simulink model "CtrPlatform"  (Simulink 7.9)
settings: Solver=ode3  StartTime=0.0  StopTime=8  FixedStep=Ts  RelTol=1e-3
InitFcn:
  | eval('CtrPlatformCfg')
StopFcn:
  | eval('CtrPlotTrj')
values from neighbouring files (symbols this model uses):
  A = [a1 a2 a3 a4 a5 a6]/180*pi    [Config.m]    (also in CtrPlatformCfg.m)
  a2 = 0    [Config.m]    (also in CtrPlatformCfg.m)
  a3 = 0    [Config.m]    (also in CtrPlatformCfg.m)
  a4 = 0    [Config.m]    (also in CtrPlatformCfg.m)
  a5 = 90    [Config.m]    (also in CtrPlatformCfg.m)
  a6 = 0    [Config.m]    (also in CtrPlatformCfg.m)
  Cen = Cen(:)'    [Config.m]    (also in CtrPlatformCfg.m; DynEulerTest.m = Cen'; EfDynCAD.m = [cen1,cen2,cen3,cen4,cen5,cen6]')
  CurPulseFreq = 0.25*2*pi    (= 1.57079632679)    [Config.m]    (also in CtrPlatformCfg.m)
  Deg2Rad = pi/180    (= 0.0174532925199)    [Config.m]    (also in CtrPlatformCfg.m)
  DisturbSelect = 2    [Config.m]    (also in CtrPlatformCfg.m)
  DynTrjMode = 3    [Config.m]    (also in CtrPlatformCfg.m = 1)
  FbDisturbSelect = 2    [Config.m]    (also in CtrPlatformCfg.m)
  freq = tvel/radius    (= 1)    [Config.m]    (also in CtrPlatformCfg.m)
  FrictionSelect = 2    [CtrPlatformCfg.m]
  Gravity = 9.8    [Config.m]    (also in CtrPlatformCfg.m)
  Ie1 = in1(:)'    [Config.m]    (also in CtrPlatformCfg.m; DynEulerTest.m = in1(:); EfDynCAD.m = in1(:))
  Ie2 = in2(:)'    [Config.m]    (also in CtrPlatformCfg.m; DynEulerTest.m = in2(:); EfDynCAD.m = in2(:))
  Ie3 = in3(:)'    [Config.m]    (also in CtrPlatformCfg.m; DynEulerTest.m = in3(:); EfDynCAD.m = in3(:))
  Ie4 = in4(:)'    [Config.m]    (also in CtrPlatformCfg.m; DynEulerTest.m = in4(:); EfDynCAD.m = in4(:))
  Ie5 = in5(:)'    [Config.m]    (also in CtrPlatformCfg.m; DynEulerTest.m = in5(:); EfDynCAD.m = in5(:))
  Ie6 = in6(:)'    [Config.m]    (also in CtrPlatformCfg.m; DynEulerTest.m = in6(:); EfDynCAD.m = in6(:))
  in1 = [5.2954 -0.2565 -0.6366;-0.2565 4.7000 0.2830;-0.6366 0.2829 5.8635]    [Config.m]    (also in CtrPlatformCfg.m; DynEulerTest.m; EfDynCAD.m = [0.54  -0.01 0.23)
  in2 = [5.8840 0.0072 0.0135;0.0072 6.0178 -0.1907;0.0135 -0.1907 0.3374]    [Config.m]    (also in CtrPlatformCfg.m; DynEulerTest.m; EfDynCAD.m = (R_x*R_z)*in2*(R_x*R_z)')
  in3 = [1.8201 -0.2274 -0.3112;-0.2274 2.2537 -0.1441;-0.3112 -0.1441 1.9485]    [Config.m]    (also in CtrPlatformCfg.m; DynEulerTest.m; EfDynCAD.m = (R_x*R_z)*in3*(R_x*R_z)')
  in4 = [0.0607 -0.0922 0;-0.0922 1.4493 0;0 0 1.4620]    [Config.m]    (also in CtrPlatformCfg.m; DynEulerTest.m = [0.0607 -0.0922 0;-0.0922 1.4493 0;0 0,1.4620]; EfDynCAD.m = (R_y*Rz)*in4*(R_y*Rz)')
  in5 = [0.0191 0.0032 0;0.0032 0.0228 0;0 0 0.0291]    [Config.m]    (also in CtrPlatformCfg.m; DynEulerTest.m; EfDynCAD.m = (R_x*R_y)*in5*(R_x*R_y)')
  in6 = [0.0012 0 0;0 0.0007 0;0 0 0.0007]    [Config.m]    (also in CtrPlatformCfg.m; DynEulerTest.m; EfDynCAD.m = (R_y*Rz)*in6*(R_y*Rz)')
  init_Endx = gd_init(1,4)    [Config.m]    (also in CtrPlatformCfg.m)
  init_Endy = gd_init(2,4)    [Config.m]    (also in CtrPlatformCfg.m)
  init_Endz = gd_init(3,4)    [Config.m]    (also in CtrPlatformCfg.m)
  init_Rot = gd_init(1:3,1:3)    [Config.m]    (also in CtrPlatformCfg.m)
  JntOffset1 = A(1)    [Config.m]    (also in CtrPlatformCfg.m)
  JntOffset2 = A(2)    [Config.m]    (also in CtrPlatformCfg.m)
  JntOffset3 = A(3)    [Config.m]    (also in CtrPlatformCfg.m)
  JntOffset4 = A(4)    [Config.m]    (also in CtrPlatformCfg.m)
  JntOffset5 = A(5)    [Config.m]    (also in CtrPlatformCfg.m)
  JntOffset6 = A(6)    [Config.m]    (also in CtrPlatformCfg.m)
  L = [l1 l2 l3 l4 l5 l6 l7 l8 l9]    [Config.m]    (also in CtrPlatformCfg.m)
  LinePTs2RadpS = 2*pi/(EncRes*Ts)./Gear    [Config.m]    (also in CtrPlatformCfg.m)
  LinePTs2Rpm = 60/(EncRes*Ts)    (= 7.32421875)    [Config.m]    (also in CtrPlatformCfg.m)
  Ma = [ma1 ma2 ma3 ma4 ma5 ma6]    [Config.m]    (also in CtrPlatformCfg.m; DynEulerTest.m = [ma1; ma2; ma3; ma4; ma5; ma6]; EfDynCAD.m = [ma1 ma2 ma3 ma4 ma5 ma6]')
  ma1 = 170.31    [Config.m]    (also in CtrPlatformCfg.m; DynEulerTest.m; EfDynCAD.m = 77.75)
  ma2 = 63.74    [Config.m]    (also in CtrPlatformCfg.m; DynEulerTest.m; EfDynCAD.m = 32.31)
  ma3 = 98.98    [Config.m]    (also in CtrPlatformCfg.m; DynEulerTest.m; EfDynCAD.m = 18.61)
  ma4 = 24.46    [Config.m]    (also in CtrPlatformCfg.m; DynEulerTest.m; EfDynCAD.m = 15.65)
  ma5 = 5.24    [Config.m]    (also in CtrPlatformCfg.m; DynEulerTest.m; EfDynCAD.m = 3.32)
  ma6 = 0.6    [Config.m]    (also in CtrPlatformCfg.m; DynEulerTest.m; EfDynCAD.m)
  PosPulseEnable = 1    [Config.m]    (also in CtrPlatformCfg.m)
  PosVelPulseGain = 500    [Config.m]    (also in CtrPlatformCfg.m)
  Rad2Line = Gear*EncRes/(2*pi)    [Config.m]    (also in CtrPlatformCfg.m)
  Rpm2LinePTs = EncRes*Ts/60    (= 0.136533333333)    [Config.m]    (also in CtrPlatformCfg.m)
  TrajSwitch = 1    [Config.m]    (also in CtrPlatformCfg.m)
  Trq2Cur = Trq2Cur./Cur2Trq    [Config.m]    (also in CtrPlatformCfg.m)
  Ts = 1/FrHz    (= 0.00025)    [Config.m]    (also in CtrPlatformCfg.m)
  Ts_Dyn = Ts    (= 0.00025)    [Config.m]    (also in CtrPlatformCfg.m)
  tvel = 120    [Config.m]    (also in CtrPlatformCfg.m)
  VelLpAxisNum = 1    [Config.m]    (also in CtrPlatformCfg.m)
  VelPulseEnable = 0    [Config.m]    (also in CtrPlatformCfg.m)
  VelPulseGain = 500    [Config.m]    (also in CtrPlatformCfg.m)
  Volt2Trq = Volt2Trq./Trq2Cur    [Config.m]    (also in CtrPlatformCfg.m)
undefined symbols (not defined in the file or in its folder): a1, DiscIntNeverNeededParam, RobotAxis
libraries: simulink x85, mblibv1 x35, powerlib_extras x25, commnoisgen2 x2
(part 2 of 5)

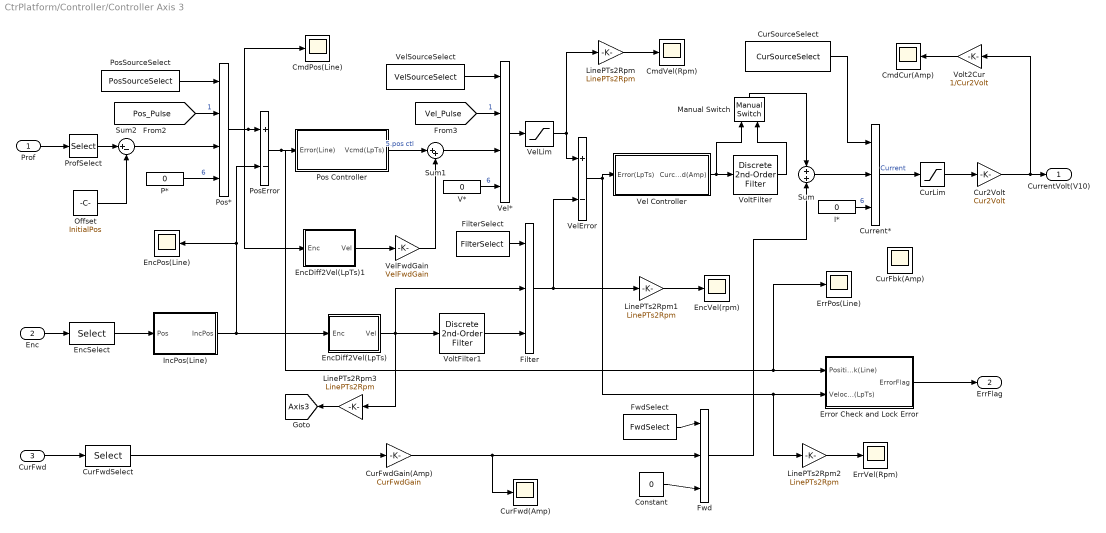
== system CtrPlatform/Controller/Controller Axis 3 ==
  Prof : Inport
  Enc : Inport  Port=2
  CurFwd : Inport  Port=3
  CmdCur(Amp) : Scope
      settings: SaveName=ScopeData42
  CmdPos(Line) : Scope
      settings: SaveName=ScopeData40
  CmdVel(Rpm) : Scope
      settings: SaveName=ScopeData39
  Constant : Constant  Value=0
  Cur2Volt : Gain  Gain=Cur2Volt  SampleTime=Ts
  CurFbk(Amp) : Scope
      settings: SaveName=ScopeData27
  CurFwd(Amp) : Scope
      settings: TimeRange=5  YMin=-600  YMax=600  SaveName=ScopeData14
  CurFwdGain(Amp) : Gain  Gain=CurFwdGain
  CurFwdSelect : Selector  InputPortWidth=6  IndexOptions=Index vector (dialog)  Indices=AxisNO  OutputSizes=1
  CurLim : Saturate  UpperLimit=CurLimit  LowerLimit=-CurLimit  SampleTime=Ts
  CurSourceSelect : Constant  Value=CurSourceSelect  SampleTime=Ts
  Current* : MultiPortSwitch  Inputs=2  zeroidx=off
  EncDiff2Vel(LpTs) : Subsystem
  EncDiff2Vel(LpTs)1 : Subsystem
  EncPos(Line) : Scope
      settings: SaveName=ScopeData41
  "EncSelect " : Selector  InputPortWidth=6  IndexOptions=Index vector (dialog)  Indices=AxisNO  OutputSizes=1
  EncVel(rpm) : Scope
      settings: SaveName=ScopeData43
  ErrPos(Line) : Scope
      settings: SaveName=ScopeData44
  ErrVel(Rpm) : Scope
      settings: SaveName=ScopeData45
  Error Check and Lock Error : Subsystem
  Filter : MultiPortSwitch  Inputs=2  zeroidx=off
  FilterSelect : Constant  Value=FilterSelect  SampleTime=Ts
  Fwd : MultiPortSwitch  Inputs=2  zeroidx=off
  FwdSelect : Constant  Value=FwdSelect  SampleTime=Ts
  I* : Constant  Value=0  SampleTime=Ts
  IncPos(Line) : Subsystem
  LinePTs2Rpm{,1..3} (4 alike) : Gain  Gain=LinePTs2Rpm
  Manual Switch : simulink/Signal Routing/Manual Switch  sw=1  action=0  varsize=off
  Offset : Constant  Value=InitialPos  SampleTime=-1
  P* : Constant  Value=0  SampleTime=Ts
  Pos Controller : Subsystem  mask{Kp=Kpp, Ki=Kpi, Kd=Kpd, Ts=Ts}
      mask prompts: Ts "Sample Time"
  Pos* : MultiPortSwitch  zeroidx=off
  PosError : Sum  Inputs=+-
  PosSourceSelect : Constant  Value=PosSourceSelect  SampleTime=Ts
  ProfSelect : Selector  InputPortWidth=6  IndexOptions=Index vector (dialog)  Indices=AxisNO  OutputSizes=1
  Sum : Sum  Inputs=+|+
  Sum1 : Sum  Inputs=|++
  Sum2 : Sum  Inputs=|+-
  V* : Constant  Value=0  SampleTime=Ts
  Vel Controller : Subsystem  mask{Kp=Kvp, Ki=Kvi, Kd=Kvd, Ts=Ts}
      mask prompts: Ts "Sample Time"
  Vel* : MultiPortSwitch  zeroidx=off
  VelError : Sum  Inputs=+-
  VelFwdGain : Gain  Gain=VelFwdGain
  VelLim : Saturate  UpperLimit=VelLimit  LowerLimit=-VelLimit  SampleTime=Ts
  VelSourceSelect : Constant  Value=VelSourceSelect  SampleTime=Ts
  Volt2Cur : Gain  Gain=1/Cur2Volt  SampleTime=Ts
  VoltFilter : powerlib_extras/Discrete  Control Blocks/Discrete  2nd-Order Filter  FilterType=Lowpass  Fo=200  Zeta=0.707  Ts=Ts  Initialize=off  Vac_Init=[0.8 -25 60]  Vdc_Init=-0.4  PlotResponse=off  param1=[1 500 1]
  VoltFilter1 : powerlib_extras/Discrete  Control Blocks/Discrete  2nd-Order Filter  FilterType=Lowpass  Fo=200  Zeta=0.707  Ts=Ts  Initialize=off  Vac_Init=[0.8 -25 60]  Vdc_Init=-0.4  PlotResponse=off  param1=[1 500 1]
  CurrentVolt(V10) : Outport
  ErrFlag : Outport  Port=2
  tag scope: Axis3=global
  wires:
  I*/1 -> Current*/3  "6"
  EncDiff2Vel(LpTs)1/1(Vel) -> VelFwdGain/1
  VelFwdGain/1 -> Sum1/2
  Volt2Cur/1 -> CmdCur(Amp)/1
  LinePTs2Rpm2/1 -> ErrVel(Rpm)/1
  LinePTs2Rpm1/1 -> EncVel(rpm)/1
  LinePTs2Rpm/1 -> CmdVel(Rpm)/1
  Cur2Volt/1 -> Volt2Cur/1, CurrentVolt(V10)/1
  CurLim/1 -> Cur2Volt/1
  VelLim/1 -> LinePTs2Rpm/1, VelError/1
  Sum1/1 -> Vel*/3
  Pos Controller/1(Vcmd(LpTs)) -> Sum1/1  "5.pos ctl"
  CurFwdGain(Amp)/1 -> CurFwd(Amp)/1, Fwd/2
  CurFwdSelect/1 -> CurFwdGain(Amp)/1
  CurFwd/1 -> CurFwdSelect/1
  V*/1 -> Vel*/4  "6"
  [Pos_Pulse] -> Pos*/2  "1"
  P*/1 -> Pos*/4  "6"
  [Vel_Pulse] -> Vel*/2  "1"
  Pos*/1 -> PosError/1, EncDiff2Vel(LpTs)1/1(Enc), CmdPos(Line)/1
  PosSourceSelect/1 -> Pos*/1
  Vel*/1 -> VelLim/1
  "EncSelect "/1 -> IncPos(Line)/1(Pos)
  Enc/1 -> "EncSelect "/1
  Prof/1 -> ProfSelect/1
  EncDiff2Vel(LpTs)/1(Vel) -> VoltFilter1/1, Filter/2, LinePTs2Rpm3/1
  VelError/1 -> LinePTs2Rpm2/1, Error Check and Lock Error/2(VelocityCheck(LpTs)), Vel Controller/1(Error(LpTs))
  VelSourceSelect/1 -> Vel*/1
  CurSourceSelect/1 -> Current*/1
  PosError/1 -> ErrPos(Line)/1, Error Check and Lock Error/1(PositionCheck(Line)), Pos Controller/1(Error(Line))
  Current*/1 -> CurLim/1  "Current"
  Error Check and Lock Error/1(ErrorFlag) -> ErrFlag/1
  IncPos(Line)/1(IncPos) -> EncPos(Line)/1, PosError/2, EncDiff2Vel(LpTs)/1(Enc)
  ProfSelect/1 -> Sum2/1
  Sum2/1 -> Pos*/3
  Offset/1 -> Sum2/2
  Vel Controller/1(Curcmd(Amp)) -> VoltFilter/1, Manual Switch/1
  VoltFilter/1 -> Manual Switch/2
  Manual Switch/1 -> Sum/1
  Sum/1 -> Current*/2
  Fwd/1 -> Sum/2
  VoltFilter1/1 -> Filter/3
  Filter/1 -> VelError/2, LinePTs2Rpm1/1
  FilterSelect/1 -> Filter/1
  Constant/1 -> Fwd/3
  FwdSelect/1 -> Fwd/1
  LinePTs2Rpm3/1 -> [Axis3]

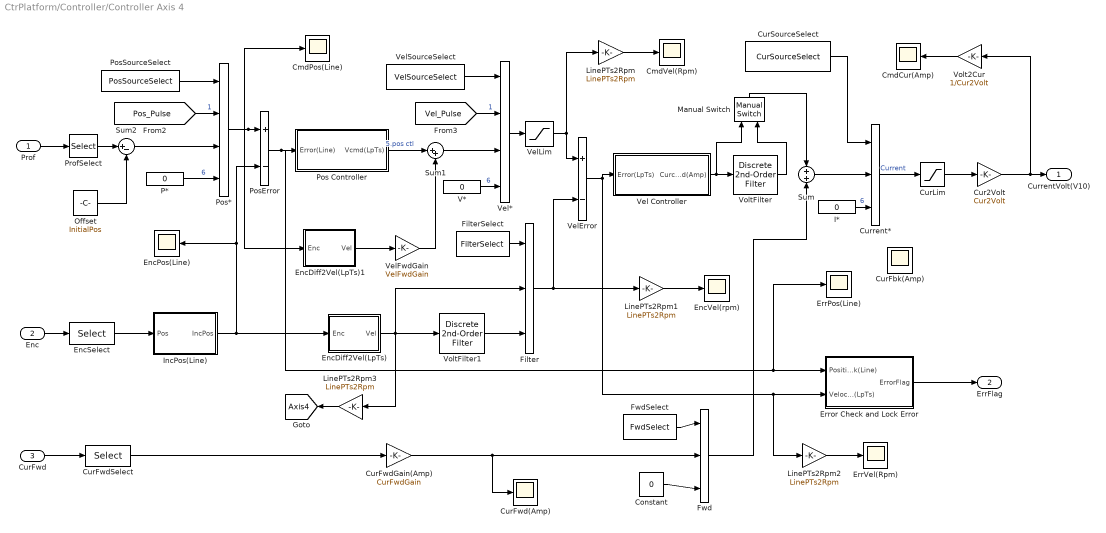
== system CtrPlatform/Controller/Controller Axis 4 ==
  Prof : Inport
  Enc : Inport  Port=2
  CurFwd : Inport  Port=3
  CmdCur(Amp) : Scope
      settings: SaveName=ScopeData42
  CmdPos(Line) : Scope
      settings: SaveName=ScopeData40
  CmdVel(Rpm) : Scope
      settings: SaveName=ScopeData39
  Constant : Constant  Value=0
  Cur2Volt : Gain  Gain=Cur2Volt  SampleTime=Ts
  CurFbk(Amp) : Scope
      settings: SaveName=ScopeData27
  CurFwd(Amp) : Scope
      settings: TimeRange=5  YMin=-600  YMax=600  SaveName=ScopeData14
  CurFwdGain(Amp) : Gain  Gain=CurFwdGain
  CurFwdSelect : Selector  InputPortWidth=6  IndexOptions=Index vector (dialog)  Indices=AxisNO  OutputSizes=1
  CurLim : Saturate  UpperLimit=CurLimit  LowerLimit=-CurLimit  SampleTime=Ts
  CurSourceSelect : Constant  Value=CurSourceSelect  SampleTime=Ts
  Current* : MultiPortSwitch  Inputs=2  zeroidx=off
  EncDiff2Vel(LpTs) : Subsystem
  EncDiff2Vel(LpTs)1 : Subsystem
  EncPos(Line) : Scope
      settings: SaveName=ScopeData41
  "EncSelect " : Selector  InputPortWidth=6  IndexOptions=Index vector (dialog)  Indices=AxisNO  OutputSizes=1
  EncVel(rpm) : Scope
      settings: SaveName=ScopeData43
  ErrPos(Line) : Scope
      settings: SaveName=ScopeData44
  ErrVel(Rpm) : Scope
      settings: SaveName=ScopeData45
  Error Check and Lock Error : Subsystem
  Filter : MultiPortSwitch  Inputs=2  zeroidx=off
  FilterSelect : Constant  Value=FilterSelect  SampleTime=Ts
  Fwd : MultiPortSwitch  Inputs=2  zeroidx=off
  FwdSelect : Constant  Value=FwdSelect  SampleTime=Ts
  I* : Constant  Value=0  SampleTime=Ts
  IncPos(Line) : Subsystem
  LinePTs2Rpm{,1..3} (4 alike) : Gain  Gain=LinePTs2Rpm
  Manual Switch : simulink/Signal Routing/Manual Switch  sw=1  action=0  varsize=off
  Offset : Constant  Value=InitialPos  SampleTime=-1
  P* : Constant  Value=0  SampleTime=Ts
  Pos Controller : Subsystem  mask{Kp=Kpp, Ki=Kpi, Kd=Kpd, Ts=Ts}
      mask prompts: Ts "Sample Time"
  Pos* : MultiPortSwitch  zeroidx=off
  PosError : Sum  Inputs=+-
  PosSourceSelect : Constant  Value=PosSourceSelect  SampleTime=Ts
  ProfSelect : Selector  InputPortWidth=6  IndexOptions=Index vector (dialog)  Indices=AxisNO  OutputSizes=1
  Sum : Sum  Inputs=+|+
  Sum1 : Sum  Inputs=|++
  Sum2 : Sum  Inputs=|+-
  V* : Constant  Value=0  SampleTime=Ts
  Vel Controller : Subsystem  mask{Kp=Kvp, Ki=Kvi, Kd=Kvd, Ts=Ts}
      mask prompts: Ts "Sample Time"
  Vel* : MultiPortSwitch  zeroidx=off
  VelError : Sum  Inputs=+-
  VelFwdGain : Gain  Gain=VelFwdGain
  VelLim : Saturate  UpperLimit=VelLimit  LowerLimit=-VelLimit  SampleTime=Ts
  VelSourceSelect : Constant  Value=VelSourceSelect  SampleTime=Ts
  Volt2Cur : Gain  Gain=1/Cur2Volt  SampleTime=Ts
  VoltFilter : powerlib_extras/Discrete  Control Blocks/Discrete  2nd-Order Filter  FilterType=Lowpass  Fo=200  Zeta=0.707  Ts=Ts  Initialize=off  Vac_Init=[0.8 -25 60]  Vdc_Init=-0.4  PlotResponse=off  param1=[1 500 1]
  VoltFilter1 : powerlib_extras/Discrete  Control Blocks/Discrete  2nd-Order Filter  FilterType=Lowpass  Fo=200  Zeta=0.707  Ts=Ts  Initialize=off  Vac_Init=[0.8 -25 60]  Vdc_Init=-0.4  PlotResponse=off  param1=[1 500 1]
  CurrentVolt(V10) : Outport
  ErrFlag : Outport  Port=2
  tag scope: Axis4=global
  wires:
  I*/1 -> Current*/3  "6"
  EncDiff2Vel(LpTs)1/1(Vel) -> VelFwdGain/1
  VelFwdGain/1 -> Sum1/2
  Volt2Cur/1 -> CmdCur(Amp)/1
  LinePTs2Rpm2/1 -> ErrVel(Rpm)/1
  LinePTs2Rpm1/1 -> EncVel(rpm)/1
  LinePTs2Rpm/1 -> CmdVel(Rpm)/1
  Cur2Volt/1 -> Volt2Cur/1, CurrentVolt(V10)/1
  CurLim/1 -> Cur2Volt/1
  VelLim/1 -> LinePTs2Rpm/1, VelError/1
  Sum1/1 -> Vel*/3
  Pos Controller/1(Vcmd(LpTs)) -> Sum1/1  "5.pos ctl"
  CurFwdGain(Amp)/1 -> CurFwd(Amp)/1, Fwd/2
  CurFwdSelect/1 -> CurFwdGain(Amp)/1
  CurFwd/1 -> CurFwdSelect/1
  V*/1 -> Vel*/4  "6"
  [Pos_Pulse] -> Pos*/2  "1"
  P*/1 -> Pos*/4  "6"
  [Vel_Pulse] -> Vel*/2  "1"
  Pos*/1 -> PosError/1, EncDiff2Vel(LpTs)1/1(Enc), CmdPos(Line)/1
  PosSourceSelect/1 -> Pos*/1
  Vel*/1 -> VelLim/1
  "EncSelect "/1 -> IncPos(Line)/1(Pos)
  Enc/1 -> "EncSelect "/1
  Prof/1 -> ProfSelect/1
  EncDiff2Vel(LpTs)/1(Vel) -> VoltFilter1/1, Filter/2, LinePTs2Rpm3/1
  VelError/1 -> LinePTs2Rpm2/1, Error Check and Lock Error/2(VelocityCheck(LpTs)), Vel Controller/1(Error(LpTs))
  VelSourceSelect/1 -> Vel*/1
  CurSourceSelect/1 -> Current*/1
  PosError/1 -> ErrPos(Line)/1, Error Check and Lock Error/1(PositionCheck(Line)), Pos Controller/1(Error(Line))
  Current*/1 -> CurLim/1  "Current"
  Error Check and Lock Error/1(ErrorFlag) -> ErrFlag/1
  IncPos(Line)/1(IncPos) -> EncPos(Line)/1, PosError/2, EncDiff2Vel(LpTs)/1(Enc)
  ProfSelect/1 -> Sum2/1
  Sum2/1 -> Pos*/3
  Offset/1 -> Sum2/2
  Vel Controller/1(Curcmd(Amp)) -> VoltFilter/1, Manual Switch/1
  VoltFilter/1 -> Manual Switch/2
  Manual Switch/1 -> Sum/1
  Sum/1 -> Current*/2
  Fwd/1 -> Sum/2
  VoltFilter1/1 -> Filter/3
  Filter/1 -> VelError/2, LinePTs2Rpm1/1
  FilterSelect/1 -> Filter/1
  Constant/1 -> Fwd/3
  FwdSelect/1 -> Fwd/1
  LinePTs2Rpm3/1 -> [Axis4]

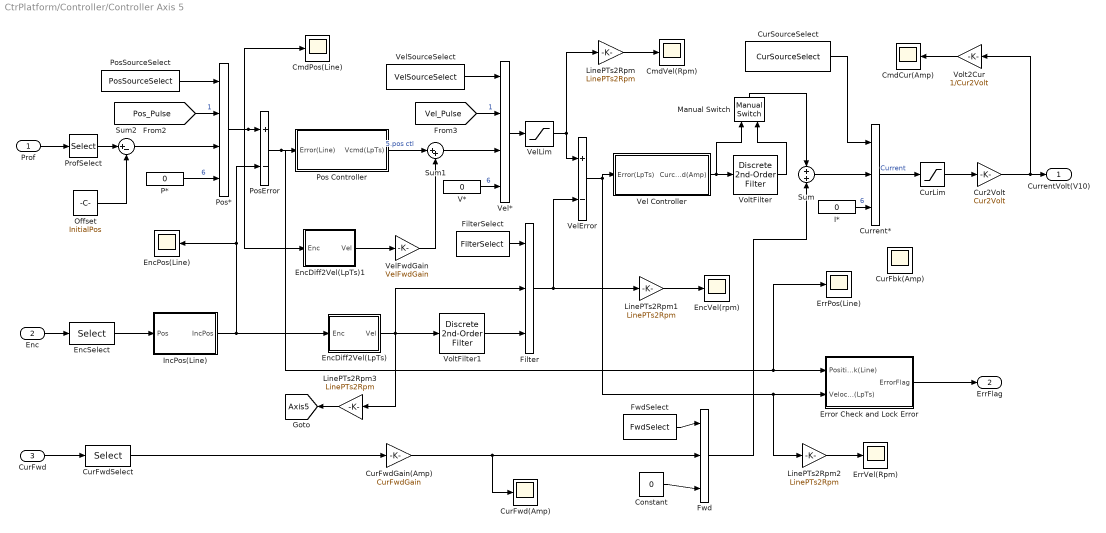
== system CtrPlatform/Controller/Controller Axis 5 ==
  Prof : Inport
  Enc : Inport  Port=2
  CurFwd : Inport  Port=3
  CmdCur(Amp) : Scope
      settings: SaveName=ScopeData42
  CmdPos(Line) : Scope
      settings: SaveName=ScopeData40
  CmdVel(Rpm) : Scope
      settings: SaveName=ScopeData39
  Constant : Constant  Value=0
  Cur2Volt : Gain  Gain=Cur2Volt  SampleTime=Ts
  CurFbk(Amp) : Scope
      settings: SaveName=ScopeData27
  CurFwd(Amp) : Scope
      settings: TimeRange=5  YMin=-600  YMax=600  SaveName=ScopeData14
  CurFwdGain(Amp) : Gain  Gain=CurFwdGain
  CurFwdSelect : Selector  InputPortWidth=6  IndexOptions=Index vector (dialog)  Indices=AxisNO  OutputSizes=1
  CurLim : Saturate  UpperLimit=CurLimit  LowerLimit=-CurLimit  SampleTime=Ts
  CurSourceSelect : Constant  Value=CurSourceSelect  SampleTime=Ts
  Current* : MultiPortSwitch  Inputs=2  zeroidx=off
  EncDiff2Vel(LpTs) : Subsystem
  EncDiff2Vel(LpTs)1 : Subsystem
  EncPos(Line) : Scope
      settings: SaveName=ScopeData41
  "EncSelect " : Selector  InputPortWidth=6  IndexOptions=Index vector (dialog)  Indices=AxisNO  OutputSizes=1
  EncVel(rpm) : Scope
      settings: SaveName=ScopeData43
  ErrPos(Line) : Scope
      settings: SaveName=ScopeData44
  ErrVel(Rpm) : Scope
      settings: SaveName=ScopeData45
  Error Check and Lock Error : Subsystem
  Filter : MultiPortSwitch  Inputs=2  zeroidx=off
  FilterSelect : Constant  Value=FilterSelect  SampleTime=Ts
  Fwd : MultiPortSwitch  Inputs=2  zeroidx=off
  FwdSelect : Constant  Value=FwdSelect  SampleTime=Ts
  I* : Constant  Value=0  SampleTime=Ts
  IncPos(Line) : Subsystem
  LinePTs2Rpm{,1..3} (4 alike) : Gain  Gain=LinePTs2Rpm
  Manual Switch : simulink/Signal Routing/Manual Switch  sw=1  action=0  varsize=off
  Offset : Constant  Value=InitialPos  SampleTime=-1
  P* : Constant  Value=0  SampleTime=Ts
  Pos Controller : Subsystem  mask{Kp=Kpp, Ki=Kpi, Kd=Kpd, Ts=Ts}
      mask prompts: Ts "Sample Time"
  Pos* : MultiPortSwitch  zeroidx=off
  PosError : Sum  Inputs=+-
  PosSourceSelect : Constant  Value=PosSourceSelect  SampleTime=Ts
  ProfSelect : Selector  InputPortWidth=6  IndexOptions=Index vector (dialog)  Indices=AxisNO  OutputSizes=1
  Sum : Sum  Inputs=+|+
  Sum1 : Sum  Inputs=|++
  Sum2 : Sum  Inputs=|+-
  V* : Constant  Value=0  SampleTime=Ts
  Vel Controller : Subsystem  mask{Kp=Kvp, Ki=Kvi, Kd=Kvd, Ts=Ts}
      mask prompts: Ts "Sample Time"
  Vel* : MultiPortSwitch  zeroidx=off
  VelError : Sum  Inputs=+-
  VelFwdGain : Gain  Gain=VelFwdGain
  VelLim : Saturate  UpperLimit=VelLimit  LowerLimit=-VelLimit  SampleTime=Ts
  VelSourceSelect : Constant  Value=VelSourceSelect  SampleTime=Ts
  Volt2Cur : Gain  Gain=1/Cur2Volt  SampleTime=Ts
  VoltFilter : powerlib_extras/Discrete  Control Blocks/Discrete  2nd-Order Filter  FilterType=Lowpass  Fo=200  Zeta=0.707  Ts=Ts  Initialize=off  Vac_Init=[0.8 -25 60]  Vdc_Init=-0.4  PlotResponse=off  param1=[1 500 1]
  VoltFilter1 : powerlib_extras/Discrete  Control Blocks/Discrete  2nd-Order Filter  FilterType=Lowpass  Fo=200  Zeta=0.707  Ts=Ts  Initialize=off  Vac_Init=[0.8 -25 60]  Vdc_Init=-0.4  PlotResponse=off  param1=[1 500 1]
  CurrentVolt(V10) : Outport
  ErrFlag : Outport  Port=2
  tag scope: Axis5=global
  wires:
  I*/1 -> Current*/3  "6"
  EncDiff2Vel(LpTs)1/1(Vel) -> VelFwdGain/1
  VelFwdGain/1 -> Sum1/2
  Volt2Cur/1 -> CmdCur(Amp)/1
  LinePTs2Rpm2/1 -> ErrVel(Rpm)/1
  LinePTs2Rpm1/1 -> EncVel(rpm)/1
  LinePTs2Rpm/1 -> CmdVel(Rpm)/1
  Cur2Volt/1 -> Volt2Cur/1, CurrentVolt(V10)/1
  CurLim/1 -> Cur2Volt/1
  VelLim/1 -> LinePTs2Rpm/1, VelError/1
  Sum1/1 -> Vel*/3
  Pos Controller/1(Vcmd(LpTs)) -> Sum1/1  "5.pos ctl"
  CurFwdGain(Amp)/1 -> CurFwd(Amp)/1, Fwd/2
  CurFwdSelect/1 -> CurFwdGain(Amp)/1
  CurFwd/1 -> CurFwdSelect/1
  V*/1 -> Vel*/4  "6"
  [Pos_Pulse] -> Pos*/2  "1"
  P*/1 -> Pos*/4  "6"
  [Vel_Pulse] -> Vel*/2  "1"
  Pos*/1 -> PosError/1, EncDiff2Vel(LpTs)1/1(Enc), CmdPos(Line)/1
  PosSourceSelect/1 -> Pos*/1
  Vel*/1 -> VelLim/1
  "EncSelect "/1 -> IncPos(Line)/1(Pos)
  Enc/1 -> "EncSelect "/1
  Prof/1 -> ProfSelect/1
  EncDiff2Vel(LpTs)/1(Vel) -> VoltFilter1/1, Filter/2, LinePTs2Rpm3/1
  VelError/1 -> LinePTs2Rpm2/1, Error Check and Lock Error/2(VelocityCheck(LpTs)), Vel Controller/1(Error(LpTs))
  VelSourceSelect/1 -> Vel*/1
  CurSourceSelect/1 -> Current*/1
  PosError/1 -> ErrPos(Line)/1, Error Check and Lock Error/1(PositionCheck(Line)), Pos Controller/1(Error(Line))
  Current*/1 -> CurLim/1  "Current"
  Error Check and Lock Error/1(ErrorFlag) -> ErrFlag/1
  IncPos(Line)/1(IncPos) -> EncPos(Line)/1, PosError/2, EncDiff2Vel(LpTs)/1(Enc)
  ProfSelect/1 -> Sum2/1
  Sum2/1 -> Pos*/3
  Offset/1 -> Sum2/2
  Vel Controller/1(Curcmd(Amp)) -> VoltFilter/1, Manual Switch/1
  VoltFilter/1 -> Manual Switch/2
  Manual Switch/1 -> Sum/1
  Sum/1 -> Current*/2
  Fwd/1 -> Sum/2
  VoltFilter1/1 -> Filter/3
  Filter/1 -> VelError/2, LinePTs2Rpm1/1
  FilterSelect/1 -> Filter/1
  Constant/1 -> Fwd/3
  FwdSelect/1 -> Fwd/1
  LinePTs2Rpm3/1 -> [Axis5]

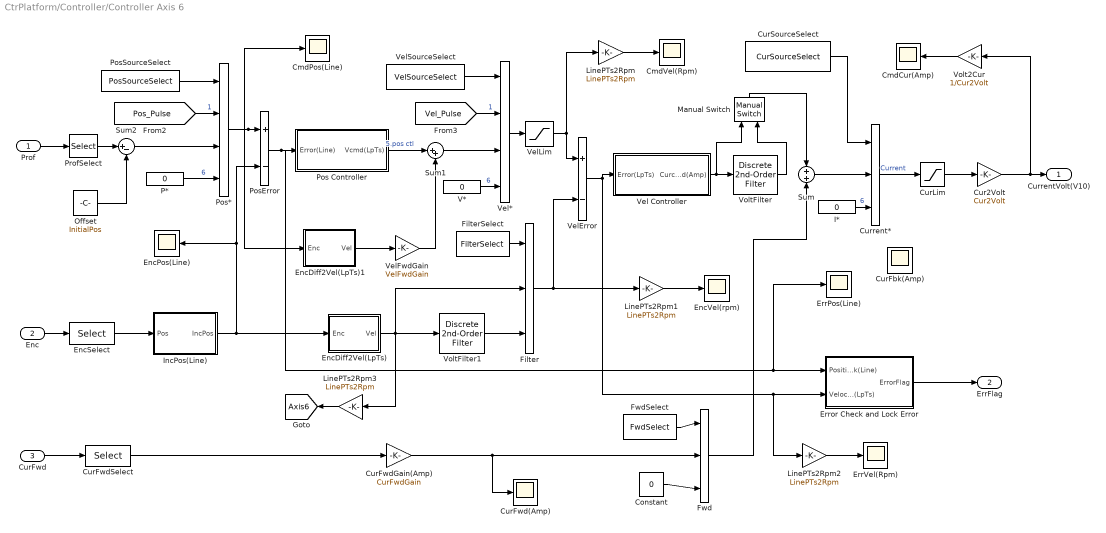
== system CtrPlatform/Controller/Controller Axis 6 ==
  Prof : Inport
  Enc : Inport  Port=2
  CurFwd : Inport  Port=3
  CmdCur(Amp) : Scope
      settings: SaveName=ScopeData42
  CmdPos(Line) : Scope
      settings: SaveName=ScopeData40
  CmdVel(Rpm) : Scope
      settings: SaveName=ScopeData39
  Constant : Constant  Value=0
  Cur2Volt : Gain  Gain=Cur2Volt  SampleTime=Ts
  CurFbk(Amp) : Scope
      settings: SaveName=ScopeData27
  CurFwd(Amp) : Scope
      settings: TimeRange=5  YMin=-600  YMax=600  SaveName=ScopeData14
  CurFwdGain(Amp) : Gain  Gain=CurFwdGain
  CurFwdSelect : Selector  InputPortWidth=6  IndexOptions=Index vector (dialog)  Indices=AxisNO  OutputSizes=1
  CurLim : Saturate  UpperLimit=CurLimit  LowerLimit=-CurLimit  SampleTime=Ts
  CurSourceSelect : Constant  Value=CurSourceSelect  SampleTime=Ts
  Current* : MultiPortSwitch  Inputs=2  zeroidx=off
  EncDiff2Vel(LpTs) : Subsystem
  EncDiff2Vel(LpTs)1 : Subsystem
  EncPos(Line) : Scope
      settings: SaveName=ScopeData41
  "EncSelect " : Selector  InputPortWidth=6  IndexOptions=Index vector (dialog)  Indices=AxisNO  OutputSizes=1
  EncVel(rpm) : Scope
      settings: SaveName=ScopeData43
  ErrPos(Line) : Scope
      settings: SaveName=ScopeData44
  ErrVel(Rpm) : Scope
      settings: SaveName=ScopeData45
  Error Check and Lock Error : Subsystem
  Filter : MultiPortSwitch  Inputs=2  zeroidx=off
  FilterSelect : Constant  Value=FilterSelect  SampleTime=Ts
  Fwd : MultiPortSwitch  Inputs=2  zeroidx=off
  FwdSelect : Constant  Value=FwdSelect  SampleTime=Ts
  I* : Constant  Value=0  SampleTime=Ts
  IncPos(Line) : Subsystem
  LinePTs2Rpm{,1..3} (4 alike) : Gain  Gain=LinePTs2Rpm
  Manual Switch : simulink/Signal Routing/Manual Switch  sw=1  action=0  varsize=off
  Offset : Constant  Value=InitialPos  SampleTime=-1
  P* : Constant  Value=0  SampleTime=Ts
  Pos Controller : Subsystem  mask{Kp=Kpp, Ki=Kpi, Kd=Kpd, Ts=Ts}
      mask prompts: Ts "Sample Time"
  Pos* : MultiPortSwitch  zeroidx=off
  PosError : Sum  Inputs=+-
  PosSourceSelect : Constant  Value=PosSourceSelect  SampleTime=Ts
  ProfSelect : Selector  InputPortWidth=6  IndexOptions=Index vector (dialog)  Indices=AxisNO  OutputSizes=1
  Sum : Sum  Inputs=+|+
  Sum1 : Sum  Inputs=|++
  Sum2 : Sum  Inputs=|+-
  V* : Constant  Value=0  SampleTime=Ts
  Vel Controller : Subsystem  mask{Kp=Kvp, Ki=Kvi, Kd=Kvd, Ts=Ts}
      mask prompts: Ts "Sample Time"
  Vel* : MultiPortSwitch  zeroidx=off
  VelError : Sum  Inputs=+-
  VelFwdGain : Gain  Gain=VelFwdGain
  VelLim : Saturate  UpperLimit=VelLimit  LowerLimit=-VelLimit  SampleTime=Ts
  VelSourceSelect : Constant  Value=VelSourceSelect  SampleTime=Ts
  Volt2Cur : Gain  Gain=1/Cur2Volt  SampleTime=Ts
  VoltFilter : powerlib_extras/Discrete  Control Blocks/Discrete  2nd-Order Filter  FilterType=Lowpass  Fo=200  Zeta=0.707  Ts=Ts  Initialize=off  Vac_Init=[0.8 -25 60]  Vdc_Init=-0.4  PlotResponse=off  param1=[1 500 1]
  VoltFilter1 : powerlib_extras/Discrete  Control Blocks/Discrete  2nd-Order Filter  FilterType=Lowpass  Fo=200  Zeta=0.707  Ts=Ts  Initialize=off  Vac_Init=[0.8 -25 60]  Vdc_Init=-0.4  PlotResponse=off  param1=[1 500 1]
  CurrentVolt(V10) : Outport
  ErrFlag : Outport  Port=2
  tag scope: Axis6=global
  wires:
  I*/1 -> Current*/3  "6"
  EncDiff2Vel(LpTs)1/1(Vel) -> VelFwdGain/1
  VelFwdGain/1 -> Sum1/2
  Volt2Cur/1 -> CmdCur(Amp)/1
  LinePTs2Rpm2/1 -> ErrVel(Rpm)/1
  LinePTs2Rpm1/1 -> EncVel(rpm)/1
  LinePTs2Rpm/1 -> CmdVel(Rpm)/1
  Cur2Volt/1 -> Volt2Cur/1, CurrentVolt(V10)/1
  CurLim/1 -> Cur2Volt/1
  VelLim/1 -> LinePTs2Rpm/1, VelError/1
  Sum1/1 -> Vel*/3
  Pos Controller/1(Vcmd(LpTs)) -> Sum1/1  "5.pos ctl"
  CurFwdGain(Amp)/1 -> CurFwd(Amp)/1, Fwd/2
  CurFwdSelect/1 -> CurFwdGain(Amp)/1
  CurFwd/1 -> CurFwdSelect/1
  V*/1 -> Vel*/4  "6"
  [Pos_Pulse] -> Pos*/2  "1"
  P*/1 -> Pos*/4  "6"
  [Vel_Pulse] -> Vel*/2  "1"
  Pos*/1 -> PosError/1, EncDiff2Vel(LpTs)1/1(Enc), CmdPos(Line)/1
  PosSourceSelect/1 -> Pos*/1
  Vel*/1 -> VelLim/1
  "EncSelect "/1 -> IncPos(Line)/1(Pos)
  Enc/1 -> "EncSelect "/1
  Prof/1 -> ProfSelect/1
  EncDiff2Vel(LpTs)/1(Vel) -> VoltFilter1/1, Filter/2, LinePTs2Rpm3/1
  VelError/1 -> LinePTs2Rpm2/1, Error Check and Lock Error/2(VelocityCheck(LpTs)), Vel Controller/1(Error(LpTs))
  VelSourceSelect/1 -> Vel*/1
  CurSourceSelect/1 -> Current*/1
  PosError/1 -> ErrPos(Line)/1, Error Check and Lock Error/1(PositionCheck(Line)), Pos Controller/1(Error(Line))
  Current*/1 -> CurLim/1  "Current"
  Error Check and Lock Error/1(ErrorFlag) -> ErrFlag/1
  IncPos(Line)/1(IncPos) -> EncPos(Line)/1, PosError/2, EncDiff2Vel(LpTs)/1(Enc)
  ProfSelect/1 -> Sum2/1
  Sum2/1 -> Pos*/3
  Offset/1 -> Sum2/2
  Vel Controller/1(Curcmd(Amp)) -> VoltFilter/1, Manual Switch/1
  VoltFilter/1 -> Manual Switch/2
  Manual Switch/1 -> Sum/1
  Sum/1 -> Current*/2
  Fwd/1 -> Sum/2
  VoltFilter1/1 -> Filter/3
  Filter/1 -> VelError/2, LinePTs2Rpm1/1
  FilterSelect/1 -> Filter/1
  Constant/1 -> Fwd/3
  FwdSelect/1 -> Fwd/1
  LinePTs2Rpm3/1 -> [Axis6]

== system CtrPlatform/Controller/Disturb ==
  Constant : Constant  Value=0  SampleTime=Ts
  DisturbSelect : Constant  Value=DisturbSelect  SampleTime=Ts
  Gaussian Noise Generator : commnoisgen2/Gaussian Noise Generator  m=0  d=0.01  s=41  Ts=Ts  frameBased=off  sampPerFrame=1  orient=off  outDataType=double
  Multiport Switch : MultiPortSwitch  Inputs=2  zeroidx=off
  Disturb : Outport
  wires:
  Gaussian Noise Generator/1 -> Multiport Switch/2
  DisturbSelect/1 -> Multiport Switch/1
  Multiport Switch/1 -> Disturb/1
  Constant/1 -> Multiport Switch/3

== system CtrPlatform/Controller/Source Model ==
  Int : DiscreteTransferFcn  Numerator=[1 0]  Denominator=[1 -1]  SampleTime=Ts
  Pos Pulse Enable : Constant  Value=PosPulseEnable  OutDataTypeStr=boolean  SampleTime=Ts_Dyn
  PosVel Pulse Cmd : Subsystem
  Rate Transition1 : RateTransition  OutPortSampleTime=Ts
  Rate Transition2 : RateTransition  OutPortSampleTime=Ts
  Rate Transition4 : RateTransition  OutPortSampleTime=Ts
  RefPosPulse : ToWorkspace  VariableName=RefPosPulse  SampleTime=-1  SaveFormat=Structure
  RefPosVelPulse : ToWorkspace  VariableName=RefPosVelPulse  SampleTime=-1  SaveFormat=Structure
  RefVelPulse : ToWorkspace  VariableName=RefVelPulse  SampleTime=-1  SaveFormat=Structure
  Vel Pulse Cmd : Subsystem
  Vel Pulse Enable : Constant  Value=VelPulseEnable  OutDataTypeStr=boolean  SampleTime=Ts_Dyn
  tag scope: PosVel_Pulse_Dyn=global, Pos_Pulse=global, Vel_Pulse=global, Vel_Pulse_Dyn=global
  wires:
  PosVel Pulse Cmd/1(Cmd(LpTs)) -> [PosVel_Pulse_Dyn], Rate Transition4/1, Rate Transition2/1
  Pos Pulse Enable/1 -> PosVel Pulse Cmd/1(Enable)
  Vel Pulse Enable/1 -> Vel Pulse Cmd/1(Enable)
  Vel Pulse Cmd/1(Cmd(LpTs)) -> Rate Transition1/1, [Vel_Pulse_Dyn]
  Rate Transition1/1 -> [Vel_Pulse], RefVelPulse/1
  Int/1 -> [Pos_Pulse], RefPosPulse/1
  Rate Transition4/1 -> RefPosVelPulse/1
  Rate Transition2/1 -> Int/1

== system CtrPlatform/Display/EndTrjDisplay ==
  End : Inport
  RefEnd : Inport  Port=2
  Demux : Demux  Outputs=5
  Demux1 : Demux  Outputs=5
  EndAccDisplay : Subsystem
  EndPosDisplay : Subsystem
  EndVelDisplay : Subsystem
  Mux{,1..3} (4 alike) : Mux  Inputs=2
  wires:
  End/1 -> Demux/1
  Demux/2 -> Mux/1
  Demux/3 -> Mux/2
  Demux/4 -> Mux1/1
  Demux/5 -> Mux1/2
  Demux1/2 -> Mux2/1
  Demux1/3 -> Mux2/2
  Demux1/4 -> Mux3/1
  Demux1/5 -> Mux3/2
  RefEnd/1 -> Demux1/1
  Demux/1 -> EndPosDisplay/1(EndPos)
  Demux1/1 -> EndPosDisplay/2(Ref_EndPos)
  Mux2/1 -> EndVelDisplay/2(Ref_EndVel)
  Mux1/1 -> EndAccDisplay/1(EndAcc)
  Mux3/1 -> EndAccDisplay/2(Ref_EndAcc)
  Mux/1 -> EndVelDisplay/1(EndVel)

== system CtrPlatform/Display/JntVelAccDisplay ==
  JointVelAcc : Inport
  Ref_JntVelAcc : Inport  Port=2
  Demux1 : Demux  Outputs=6
  Demux3 : Demux  Outputs=6
  Joint1 : Subsystem
  Joint2 : Subsystem
  Joint3 : Subsystem
  Joint4 : Subsystem
  Joint5 : Subsystem
  Joint6 : Subsystem
  Volt2Trq : Gain
  Volt2Trq1 : Gain
  wires:
  Demux1/6 -> Joint6/2(Ref_JVA6)
  Demux3/6 -> Joint6/1(JVA6)
  Demux1/5 -> Joint5/2(Ref_JVA5)
  Demux3/5 -> Joint5/1(JVA5)
  Demux1/4 -> Joint4/2(Ref_JVA4)
  Demux3/4 -> Joint4/1(JVA4)
  Demux1/3 -> Joint3/2(Ref_JVA3)
  Demux3/3 -> Joint3/1(JVA3)
  Demux1/2 -> Joint2/2(Ref_JVA2)
  Demux3/2 -> Joint2/1(JVA2)
  Demux3/1 -> Joint1/1(JVA1)
  Demux1/1 -> Joint1/2(Ref_JVA1)
  Ref_JntVelAcc/1 -> Volt2Trq1/1
  JointVelAcc/1 -> Volt2Trq/1
  Volt2Trq/1 -> Demux3/1
  Volt2Trq1/1 -> Demux1/1

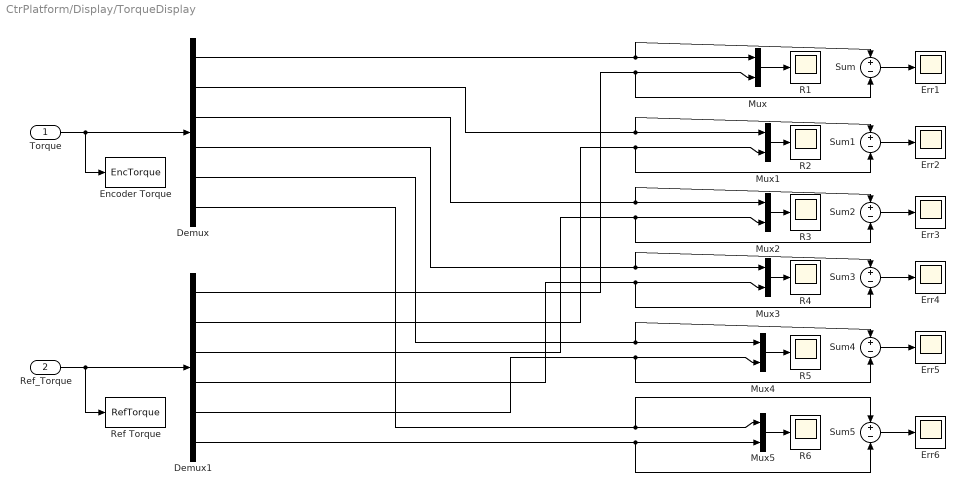
== system CtrPlatform/Display/TorqueDisplay ==
  Torque : Inport
  Ref_Torque : Inport  Port=2
  Demux : Demux  Outputs=6
  Demux1 : Demux  Outputs=6
  Encoder Torque : ToWorkspace  VariableName=EncTorque  SampleTime=-1  SaveFormat=Structure
  Err{1..6} (6 alike) : Scope
      Err1 settings: SaveName=ScopeData6
      Err2 settings: SaveName=ScopeData7
      Err3 settings: SaveName=ScopeData8
      Err4 settings: SaveName=ScopeData9
      Err5 settings: TimeRange=3  YMin=-2.5  YMax=1  SaveName=ScopeData10
      Err6 settings: SaveName=ScopeData11
  Mux{,1..5} (6 alike) : Mux  Inputs=2
  R{1..6} (6 alike) : Scope
      R1 settings: SaveName=ScopeData29
      R2 settings: TimeRange=10  YMin=-3e-17  YMax=4e-17  SaveName=ScopeData34
      R3 settings: SaveName=ScopeData35
      R4 settings: SaveName=ScopeData46
      R5 settings: TimeRange=10  YMin=-4.18  YMax=-4.04  SaveName=ScopeData47
      R6 settings: TimeRange=10  YMin=-1.6e-06  YMax=4e-07  SaveName=ScopeData48
  Ref Torque : ToWorkspace  VariableName=RefTorque  SampleTime=-1  SaveFormat=Structure
  Sum{,1..5} (6 alike) : Sum  Inputs=+|-
  wires:
  Sum/1 -> Err1/1
  Sum1/1 -> Err2/1
  Sum2/1 -> Err3/1
  Sum3/1 -> Err4/1
  Sum4/1 -> Err5/1
  Sum5/1 -> Err6/1
  Torque/1 -> Demux/1, Encoder Torque/1
  Ref_Torque/1 -> Demux1/1, Ref Torque/1
  Demux/1 -> Sum/1, Mux/1
  Demux1/1 -> Sum/2, Mux/2
  Demux/2 -> Sum1/1, Mux1/1
  Demux/3 -> Sum2/1, Mux2/1
  Demux/4 -> Sum3/1, Mux3/1
  Demux/5 -> Sum4/1, Mux4/1
  Demux/6 -> Sum5/1, Mux5/1
  Demux1/2 -> Sum1/2, Mux1/2
  Demux1/3 -> Sum2/2, Mux2/2
  Demux1/4 -> Sum3/2, Mux3/2
  Demux1/5 -> Sum4/2, Mux4/2
  Demux1/6 -> Sum5/2, Mux5/2
  Mux/1 -> R1/1
  Mux1/1 -> R2/1
  Mux2/1 -> R3/1
  Mux3/1 -> R4/1
  Mux4/1 -> R5/1
  Mux5/1 -> R6/1

== system CtrPlatform/Dynamics/C_Omega Display ==
  C_Omega : Inport
  Demux : Demux  Outputs=6
  Jnt{1..6} (6 alike) : Scope
      Jnt1 settings: SaveName=ScopeData19
      Jnt2 settings: SaveName=ScopeData20
      Jnt3 settings: SaveName=ScopeData22
      Jnt4 settings: SaveName=ScopeData23
      Jnt5 settings: SaveName=ScopeData24
      Jnt6 settings: SaveName=ScopeData25
  wires:
  C_Omega/1 -> Demux/1
  Demux/1 -> Jnt1/1
  Demux/2 -> Jnt2/1
  Demux/3 -> Jnt3/1
  Demux/4 -> Jnt4/1
  Demux/5 -> Jnt5/1
  Demux/6 -> Jnt6/1

== system CtrPlatform/Dynamics/M_Acc Display ==
  M_Acc : Inport
  Demux : Demux  Outputs=6
  Jnt{1..6} (6 alike) : Scope
      Jnt1 settings: SaveName=ScopeData19
      Jnt2 settings: SaveName=ScopeData20
      Jnt3 settings: SaveName=ScopeData22
      Jnt4 settings: SaveName=ScopeData23
      Jnt5 settings: SaveName=ScopeData24
      Jnt6 settings: SaveName=ScopeData25
  wires:
  M_Acc/1 -> Demux/1
  Demux/1 -> Jnt1/1
  Demux/2 -> Jnt2/1
  Demux/3 -> Jnt3/1
  Demux/4 -> Jnt4/1
  Demux/5 -> Jnt5/1
  Demux/6 -> Jnt6/1

== system CtrPlatform/Dynamics/N Display ==
  N : Inport
  Demux : Demux  Outputs=6
  Jnt{1..6} (6 alike) : Scope
      Jnt1 settings: SaveName=ScopeData19
      Jnt2 settings: SaveName=ScopeData20
      Jnt3 settings: SaveName=ScopeData22
      Jnt4 settings: SaveName=ScopeData23
      Jnt5 settings: SaveName=ScopeData24
      Jnt6 settings: SaveName=ScopeData25
  wires:
  Demux/6 -> Jnt6/1
  Demux/5 -> Jnt5/1
  Demux/4 -> Jnt4/1
  Demux/3 -> Jnt3/1
  Demux/2 -> Jnt2/1
  Demux/1 -> Jnt1/1
  N/1 -> Demux/1

== system CtrPlatform/Dynamics/Torque Display ==
  Torque : Inport
  Demux : Demux  Outputs=6
  Jnt{1..6} (6 alike) : Scope
      Jnt1 settings: SaveName=ScopeData19
      Jnt2 settings: SaveName=ScopeData20
      Jnt3 settings: SaveName=ScopeData22
      Jnt4 settings: SaveName=ScopeData23
      Jnt5 settings: SaveName=ScopeData24
      Jnt6 settings: SaveName=ScopeData25
  wires:
  Demux/6 -> Jnt6/1
  Demux/5 -> Jnt5/1
  Demux/4 -> Jnt4/1
  Demux/3 -> Jnt3/1
  Demux/2 -> Jnt2/1
  Demux/1 -> Jnt1/1
  Torque/1 -> Demux/1

== system CtrPlatform/Dynamics/TrjSource ==
  Demux : Demux  Outputs=3
  DynTrjMode : Constant  Value=DynTrjMode  SampleTime=Ts_Dyn
  Multiport Switch : MultiPortSwitch  Inputs=4  zeroidx=off
  Mux : Mux  Inputs=3
  Mux1 : Mux  Inputs=3
  Mux2 : Mux  Inputs=3
  Position Loop Tunning : Subsystem
  "Robot Profile " : Subsystem
  Velocity Loop Tunning : Subsystem
  zero : Constant  Value=zeros(1,18)
  RefJntPos(Rad) : Outport
  RefJntVel(Rad/s) : Outport  Port=2
  RefJntAcc(Rad/s2) : Outport  Port=3
  wires:
  DynTrjMode/1 -> Multiport Switch/1
  "Robot Profile "/1(JntPos(Rad)) -> Mux/1
  "Robot Profile "/2(JntVel(Rad/s)) -> Mux/2
  "Robot Profile "/3(JntAcc(Rad/s2)) -> Mux/3
  Mux/1 -> Multiport Switch/2
  Velocity Loop Tunning/1(JntPos(Rad)) -> Mux1/1
  Velocity Loop Tunning/2(JntVel(Rad/s)) -> Mux1/2
  Velocity Loop Tunning/3(JntAcc(Rad/s2)) -> Mux1/3
  Mux1/1 -> Multiport Switch/3
  Position Loop Tunning/1(JntPos(Rad)) -> Mux2/1
  Position Loop Tunning/2(JntVel(Rad/s)) -> Mux2/2
  Position Loop Tunning/3(JntAcc(Rad/s2)) -> Mux2/3
  Mux2/1 -> Multiport Switch/4
  Multiport Switch/1 -> Demux/1
  Demux/3 -> RefJntAcc(Rad/s2)/1
  Demux/2 -> RefJntVel(Rad/s)/1
  Demux/1 -> RefJntPos(Rad)/1
  zero/1 -> Multiport Switch/5

== system CtrPlatform/Fanuc/ EndSensor ==
  Avx : Scope
      settings: TimeRange=3  YMin=-150  YMax=125  SaveName=ScopeData62
  Avy : Scope
      settings: TimeRange=3  YMin=-150  YMax=125  SaveName=ScopeData63
  Avz : Scope
      settings: TimeRange=3  YMin=-150  YMax=125  SaveName=ScopeData64
  Awx : Scope
      settings: TimeRange=3  YMin=-150  YMax=125  SaveName=ScopeData65
  Awy : Scope
      settings: TimeRange=3  YMin=-150  YMax=125  SaveName=ScopeData66
  Awz : Scope
      settings: TimeRange=3  YMin=-150  YMax=125  SaveName=ScopeData67
  "Body Sensor " : mblibv1/Sensors &  Actuators/Body Sensor  UpdateFromCAD=off  PhysicalDomain=Mechanical  PortType=blob  Muxed=on  Pose=off  Angle=on  AngleUnits=deg  ArcVelocity=on  ArcVelocityUnits=deg/s  ArcAcceleration=on  ArcAccelerationUnits=deg/s^2  CoordPosition=on  CoordPositionUnits=mm  Velocity=on  VelocityUnits=mm/s  Acceleration=on  AccelerationUnits=mm/s^2  Quaternion=on  QuaternionDT=off  QuaternionDDT=off  QuaternionUnits=off  OutputVector=[1]  ActiveIO=on  Width=15  DialogClass=MechanicalSensorBlock  ReferenceFrame=Absolute (World)
  Demux5 : Demux  Outputs=15
  EndX : ToWorkspace  VariableName=EndX  SampleTime=-1  SaveFormat=Structure
  EndY : ToWorkspace  VariableName=EndY  SampleTime=-1  SaveFormat=Structure
  EndZ : ToWorkspace  VariableName=EndZ  SampleTime=-1  SaveFormat=Structure
  Vx : Scope
      settings: TimeRange=3  YMin=-150  YMax=125  SaveName=ScopeData55
  Vy : Scope
      settings: TimeRange=3  YMin=-150  YMax=125  SaveName=ScopeData57
  Vz : Scope
      settings: TimeRange=3  YMin=-150  YMax=125  SaveName=ScopeData58
  X : Scope
      settings: TimeRange=3  YMin=-150  YMax=125  SaveName=ScopeData36
  Y : Scope
      settings: TimeRange=3  YMin=-150  YMax=125  SaveName=ScopeData37
  Z : Scope
      settings: TimeRange=3  YMin=-150  YMax=125  SaveName=ScopeData38
  wx : Scope
      settings: TimeRange=3  YMin=-150  YMax=125  SaveName=ScopeData59
  wy : Scope
      settings: TimeRange=3  YMin=-150  YMax=125  SaveName=ScopeData60
  wz : Scope
      settings: TimeRange=3  YMin=-150  YMax=125  SaveName=ScopeData61
  In : PMIOPort  Port=1  Side=Left
  Out : Outport
  wires:
  "Body Sensor "/1 -> Demux5/1, Out/1
  Demux5/4 -> Vx/1
  Demux5/5 -> Vy/1
  Demux5/6 -> Vz/1
  Demux5/7 -> wx/1
  Demux5/8 -> wy/1
  Demux5/9 -> wz/1
  Demux5/10 -> Avx/1
  Demux5/11 -> Avy/1
  Demux5/12 -> Avz/1
  Demux5/13 -> Awx/1
  Demux5/14 -> Awy/1
  Demux5/15 -> Awz/1
  Demux5/1 -> EndX/1, X/1
  Demux5/2 -> EndY/1, Y/1
  Demux5/3 -> EndZ/1, Z/1
  connections:
  In/RConn1 -- "Body Sensor "/LConn1

== system CtrPlatform/Fanuc/JointSensor1 ==
  Angle Acceleration : Scope
      settings: SaveName=ScopeData32
  Angle Velocity : Scope
      settings: SaveName=ScopeData31
  Anlge : Scope
      settings: SaveName=ScopeData30
  Computed Torque : Scope
      settings: SaveName=ScopeData33
  Demux : Demux
  Sensor1 : mblibv1/Sensors &  Actuators/Joint Sensor  UpdateFromCAD=off  PhysicalDomain=Mechanical  PortType=blob  Muxed=on  Pose=off  Angle=on  AngleUnits=deg  ArcVelocity=on  ArcVelocityUnits=deg/s  ArcAcceleration=on  ArcAccelerationUnits=deg/s^2  CoordPosition=on  CoordPositionUnits=m  Velocity=off  VelocityUnits=m/s  Acceleration=off  AccelerationUnits=m/s^2  Quaternion=on  QuaternionDT=off  QuaternionDDT=off  QuaternionUnits=off  OutputVector=[1]  ActiveIO=on  Width=4  DialogClass=MechanicalSensorBlock  Primitive=R1  Force=off  ForceUnits=N  Torque=on  TorqueUnits=N*m  ReferenceFrame=Absolute (World)  ReactionSensedSide=Follower  ReactionReferenceFrame=Absolute (World)  ReactionForce=off  ReactionForceUnits=N  ReactionMoment=off  ReactionMomentUnits=N*m
  In : PMIOPort  Port=1  Side=Left
  Out : Outport
  wires:
  Demux/4 -> Computed Torque/1
  Demux/3 -> Angle Acceleration/1
  Demux/1 -> Anlge/1
  Demux/2 -> Angle Velocity/1
  Sensor1/1 -> Out/1, Demux/1
  connections:
  In/RConn1 -- Sensor1/LConn1

== system CtrPlatform/Fanuc/JointSensor2 ==
  Angle Acceleration : Scope
      settings: SaveName=ScopeData32
  Angle Velocity : Scope
      settings: SaveName=ScopeData31
  Anlge : Scope
      settings: SaveName=ScopeData30
  Computed Torque : Scope
      settings: SaveName=ScopeData33
  Demux : Demux
  Sensor1 : mblibv1/Sensors &  Actuators/Joint Sensor  UpdateFromCAD=off  PhysicalDomain=Mechanical  PortType=blob  Muxed=on  Pose=off  Angle=on  AngleUnits=deg  ArcVelocity=on  ArcVelocityUnits=deg/s  ArcAcceleration=on  ArcAccelerationUnits=deg/s^2  CoordPosition=on  CoordPositionUnits=m  Velocity=off  VelocityUnits=m/s  Acceleration=off  AccelerationUnits=m/s^2  Quaternion=on  QuaternionDT=off  QuaternionDDT=off  QuaternionUnits=off  OutputVector=[1]  ActiveIO=on  Width=4  DialogClass=MechanicalSensorBlock  Primitive=R1  Force=off  ForceUnits=N  Torque=on  TorqueUnits=N*m  ReferenceFrame=Absolute (World)  ReactionSensedSide=Follower  ReactionReferenceFrame=Absolute (World)  ReactionForce=off  ReactionForceUnits=N  ReactionMoment=off  ReactionMomentUnits=N*m
  In : PMIOPort  Port=1  Side=Left
  Out : Outport
  wires:
  Demux/4 -> Computed Torque/1
  Demux/3 -> Angle Acceleration/1
  Demux/1 -> Anlge/1
  Demux/2 -> Angle Velocity/1
  Sensor1/1 -> Out/1, Demux/1
  connections:
  In/RConn1 -- Sensor1/LConn1

== system CtrPlatform/Fanuc/JointSensor3 ==
  Angle Acceleration : Scope
      settings: SaveName=ScopeData32
  Angle Velocity : Scope
      settings: SaveName=ScopeData31
  Anlge : Scope
      settings: SaveName=ScopeData30
  Computed Torque : Scope
      settings: SaveName=ScopeData33
  Demux : Demux
  Sensor1 : mblibv1/Sensors &  Actuators/Joint Sensor  UpdateFromCAD=off  PhysicalDomain=Mechanical  PortType=blob  Muxed=on  Pose=off  Angle=on  AngleUnits=deg  ArcVelocity=on  ArcVelocityUnits=deg/s  ArcAcceleration=on  ArcAccelerationUnits=deg/s^2  CoordPosition=on  CoordPositionUnits=m  Velocity=off  VelocityUnits=m/s  Acceleration=off  AccelerationUnits=m/s^2  Quaternion=on  QuaternionDT=off  QuaternionDDT=off  QuaternionUnits=off  OutputVector=[1]  ActiveIO=on  Width=4  DialogClass=MechanicalSensorBlock  Primitive=R1  Force=off  ForceUnits=N  Torque=on  TorqueUnits=N*m  ReferenceFrame=Absolute (World)  ReactionSensedSide=Follower  ReactionReferenceFrame=Absolute (World)  ReactionForce=off  ReactionForceUnits=N  ReactionMoment=off  ReactionMomentUnits=N*m
  In : PMIOPort  Port=1  Side=Left
  Out : Outport
  wires:
  Demux/4 -> Computed Torque/1
  Demux/3 -> Angle Acceleration/1
  Demux/1 -> Anlge/1
  Demux/2 -> Angle Velocity/1
  Sensor1/1 -> Out/1, Demux/1
  connections:
  In/RConn1 -- Sensor1/LConn1

== system CtrPlatform/Fanuc/JointSensor4 ==
  Angle Acceleration : Scope
      settings: SaveName=ScopeData32
  Angle Velocity : Scope
      settings: SaveName=ScopeData31
  Anlge : Scope
      settings: SaveName=ScopeData30
  Computed Torque : Scope
      settings: SaveName=ScopeData33
  Demux : Demux
  Sensor1 : mblibv1/Sensors &  Actuators/Joint Sensor  UpdateFromCAD=off  PhysicalDomain=Mechanical  PortType=blob  Muxed=on  Pose=off  Angle=on  AngleUnits=deg  ArcVelocity=on  ArcVelocityUnits=deg/s  ArcAcceleration=on  ArcAccelerationUnits=deg/s^2  CoordPosition=on  CoordPositionUnits=m  Velocity=off  VelocityUnits=m/s  Acceleration=off  AccelerationUnits=m/s^2  Quaternion=on  QuaternionDT=off  QuaternionDDT=off  QuaternionUnits=off  OutputVector=[1]  ActiveIO=on  Width=4  DialogClass=MechanicalSensorBlock  Primitive=R1  Force=off  ForceUnits=N  Torque=on  TorqueUnits=N*m  ReferenceFrame=Absolute (World)  ReactionSensedSide=Follower  ReactionReferenceFrame=Absolute (World)  ReactionForce=off  ReactionForceUnits=N  ReactionMoment=off  ReactionMomentUnits=N*m
  In : PMIOPort  Port=1  Side=Left
  Out : Outport
  wires:
  Demux/4 -> Computed Torque/1
  Demux/3 -> Angle Acceleration/1
  Demux/1 -> Anlge/1
  Demux/2 -> Angle Velocity/1
  Sensor1/1 -> Out/1, Demux/1
  connections:
  In/RConn1 -- Sensor1/LConn1

== system CtrPlatform/Fanuc/JointSensor5 ==
  Angle Acceleration : Scope
      settings: SaveName=ScopeData32
  Angle Velocity : Scope
      settings: SaveName=ScopeData31
  Anlge : Scope
      settings: SaveName=ScopeData30
  Computed Torque : Scope
      settings: SaveName=ScopeData33
  Demux : Demux
  Sensor1 : mblibv1/Sensors &  Actuators/Joint Sensor  UpdateFromCAD=off  PhysicalDomain=Mechanical  PortType=blob  Muxed=on  Pose=off  Angle=on  AngleUnits=deg  ArcVelocity=on  ArcVelocityUnits=deg/s  ArcAcceleration=on  ArcAccelerationUnits=deg/s^2  CoordPosition=on  CoordPositionUnits=m  Velocity=off  VelocityUnits=m/s  Acceleration=off  AccelerationUnits=m/s^2  Quaternion=on  QuaternionDT=off  QuaternionDDT=off  QuaternionUnits=off  OutputVector=[1]  ActiveIO=on  Width=4  DialogClass=MechanicalSensorBlock  Primitive=R1  Force=off  ForceUnits=N  Torque=on  TorqueUnits=N*m  ReferenceFrame=Absolute (World)  ReactionSensedSide=Follower  ReactionReferenceFrame=Absolute (World)  ReactionForce=off  ReactionForceUnits=N  ReactionMoment=off  ReactionMomentUnits=N*m
  In : PMIOPort  Port=1  Side=Left
  Out : Outport
  wires:
  Demux/4 -> Computed Torque/1
  Demux/3 -> Angle Acceleration/1
  Demux/1 -> Anlge/1
  Demux/2 -> Angle Velocity/1
  Sensor1/1 -> Out/1, Demux/1
  connections:
  In/RConn1 -- Sensor1/LConn1

== system CtrPlatform/Fanuc/JointSensor6 ==
  Angle Acceleration : Scope
      settings: SaveName=ScopeData32
  Angle Velocity : Scope
      settings: SaveName=ScopeData31
  Anlge : Scope
      settings: SaveName=ScopeData30
  Computed Torque : Scope
      settings: SaveName=ScopeData33
  Demux : Demux
  Sensor1 : mblibv1/Sensors &  Actuators/Joint Sensor  UpdateFromCAD=off  PhysicalDomain=Mechanical  PortType=blob  Muxed=on  Pose=off  Angle=on  AngleUnits=deg  ArcVelocity=on  ArcVelocityUnits=deg/s  ArcAcceleration=on  ArcAccelerationUnits=deg/s^2  CoordPosition=on  CoordPositionUnits=m  Velocity=off  VelocityUnits=m/s  Acceleration=off  AccelerationUnits=m/s^2  Quaternion=on  QuaternionDT=off  QuaternionDDT=off  QuaternionUnits=off  OutputVector=[1]  ActiveIO=on  Width=4  DialogClass=MechanicalSensorBlock  Primitive=R1  Force=off  ForceUnits=N  Torque=on  TorqueUnits=N*m  ReferenceFrame=Absolute (World)  ReactionSensedSide=Follower  ReactionReferenceFrame=Absolute (World)  ReactionForce=off  ReactionForceUnits=N  ReactionMoment=off  ReactionMomentUnits=N*m
  In : PMIOPort  Port=1  Side=Left
  Out : Outport
  wires:
  Demux/4 -> Computed Torque/1
  Demux/3 -> Angle Acceleration/1
  Demux/1 -> Anlge/1
  Demux/2 -> Angle Velocity/1
  Sensor1/1 -> Out/1, Demux/1
  connections:
  In/RConn1 -- Sensor1/LConn1

== system CtrPlatform/Friction Torque/Friction Torque ==
  Ff1 : Subsystem  mask{Ts=Ts, FpSelect=2}
      mask prompts: Ts "Sampling Time"
  Ff2 : Subsystem  mask{Ts=Ts, FpSelect=2}
      mask prompts: Ts "Sampling Time"
  Ff3 : Subsystem  mask{Ts=Ts, FpSelect=2}
      mask prompts: Ts "Sampling Time"
  Ff4 : Subsystem  mask{Ts=Ts, FpSelect=1}
      mask prompts: Ts "Sampling Time"
  Ff5 : Subsystem  mask{Ts=Ts, FpSelect=1}
      mask prompts: Ts "Sampling Time"
  Ff6 : Subsystem  mask{Ts=Ts, FpSelect=1}
      mask prompts: Ts "Sampling Time"
  Mux : Mux  Inputs=6
  Scope{1..6} (6 alike) : Scope
      Scope1 settings: SaveName=ScopeData70
      Scope2 settings: SaveName=ScopeData69
      Scope3 settings: SaveName=ScopeData71
      Scope4 settings: SaveName=ScopeData72
      Scope5 settings: SaveName=ScopeData73
      Scope6 settings: SaveName=ScopeData74
  Friction Torque : Outport
  wires:
  [Axis1] -> Ff1/1(dq)
  [Axis2] -> Ff2/1(dq)
  [Axis1] -> Ff3/1(dq)
  [Axis1] -> Ff4/1(dq)
  [Axis1] -> Ff5/1(dq)
  [Axis1] -> Ff6/1(dq)
  Ff1/1(Ff) -> Mux/1, Scope1/1
  Ff2/1(Ff) -> Mux/2, Scope2/1
  Ff3/1(Ff) -> Mux/3, Scope3/1
  Ff4/1(Ff) -> Mux/4, Scope4/1
  Ff5/1(Ff) -> Mux/5, Scope5/1
  Ff6/1(Ff) -> Mux/6, Scope6/1
  Mux/1 -> Friction Torque/1

== system CtrPlatform/Signal Re-group/Re-group ==
  JntVelAcc_R1 : Inport
  Torque_R1 : Inport  Port=2
  JntVelAcc_R2 : Inport  Port=3
  Torque_R2 : Inport  Port=4
  JntVelAcc_R3 : Inport  Port=5
  Torque_R3 : Inport  Port=6
  JntVelAcc_R4 : Inport  Port=7
  Torque_R4 : Inport  Port=8
  JntVelAcc_R5 : Inport  Port=9
  Torque_R5 : Inport  Port=10
  JntVelAcc_R6 : Inport  Port=11
  Torque_R6 : Inport  Port=12
  Mux : Mux  Inputs=6
  Mux1 : Mux  Inputs=6
  JntVelAcc : Outport
  Torque : Outport  Port=2
  wires:
  JntVelAcc_R1/1 -> Mux/1
  JntVelAcc_R2/1 -> Mux/2
  JntVelAcc_R3/1 -> Mux/3
  JntVelAcc_R4/1 -> Mux/4
  JntVelAcc_R5/1 -> Mux/5
  JntVelAcc_R6/1 -> Mux/6
  Torque_R1/1 -> Mux1/1
  Torque_R2/1 -> Mux1/2
  Torque_R3/1 -> Mux1/3
  Torque_R4/1 -> Mux1/4
  Torque_R5/1 -> Mux1/5
  Torque_R6/1 -> Mux1/6
  Mux/1 -> JntVelAcc/1
  Mux1/1 -> Torque/1

== system CtrPlatform/Signal Re-group/Re-group JntVelAcc ==
  note: Joint Angle
  note: Joint Velocity
  note: Joint Acceleration
  JntVelAcc : Inport
  Demux2 : Demux  Outputs=18
  Mux : Mux  Inputs=6
  Mux1 : Mux  Inputs=6
  Mux2 : Mux  Inputs=6
  Mux3 : Mux  Inputs=3
  ReJntVelAcc : Outport
  wires:
  JntVelAcc/1 -> Demux2/1
  Demux2/1 -> Mux/1
  Demux2/2 -> Mux1/1
  Demux2/3 -> Mux2/1
  Demux2/4 -> Mux/2
  Demux2/5 -> Mux1/2
  Demux2/6 -> Mux2/2
  Demux2/7 -> Mux/3
  Demux2/8 -> Mux1/3
  Demux2/9 -> Mux2/3
  Demux2/10 -> Mux/4
  Demux2/11 -> Mux1/4
  Demux2/12 -> Mux2/4
  Demux2/13 -> Mux/5
  Demux2/14 -> Mux1/5
  Demux2/15 -> Mux2/5
  Demux2/16 -> Mux/6
  Demux2/17 -> Mux1/6
  Demux2/18 -> Mux2/6
  Mux/1 -> Mux3/1
  Mux1/1 -> Mux3/2
  Mux2/1 -> Mux3/3
  Mux3/1 -> ReJntVelAcc/1

== system CtrPlatform/Signal Re-group/Re-group_R1 ==
  In_R1 : Inport
  Demux2 : Demux
  Mux : Mux  Inputs=3
  JntVelAcc_R1 : Outport
  Torque_R1 : Outport  Port=2
  wires:
  In_R1/1 -> Demux2/1
  Demux2/1 -> Mux/1
  Demux2/2 -> Mux/2
  Demux2/3 -> Mux/3
  Demux2/4 -> Torque_R1/1
  Mux/1 -> JntVelAcc_R1/1

== system CtrPlatform/Signal Re-group/Re-group_R2 ==
  In_R2 : Inport
  Demux2 : Demux
  Mux : Mux  Inputs=3
  JntVelAcc_R2 : Outport
  Torque_R2 : Outport  Port=2
  wires:
  Mux/1 -> JntVelAcc_R2/1
  Demux2/4 -> Torque_R2/1
  Demux2/3 -> Mux/3
  Demux2/2 -> Mux/2
  Demux2/1 -> Mux/1
  In_R2/1 -> Demux2/1

== system CtrPlatform/Signal Re-group/Re-group_R3 ==
  In_R3 : Inport
  Demux2 : Demux
  Mux : Mux  Inputs=3
  JntVelAcc_R3 : Outport
  Torque_R3 : Outport  Port=2
  wires:
  In_R3/1 -> Demux2/1
  Demux2/1 -> Mux/1
  Demux2/2 -> Mux/2
  Demux2/3 -> Mux/3
  Demux2/4 -> Torque_R3/1
  Mux/1 -> JntVelAcc_R3/1

== system CtrPlatform/Signal Re-group/Re-group_R4 ==
  In_R4 : Inport
  Demux2 : Demux
  Mux : Mux  Inputs=3
  JntVelAcc_R4 : Outport
  Torque_R4 : Outport  Port=2
  wires:
  Mux/1 -> JntVelAcc_R4/1
  Demux2/4 -> Torque_R4/1
  Demux2/3 -> Mux/3
  Demux2/2 -> Mux/2
  Demux2/1 -> Mux/1
  In_R4/1 -> Demux2/1

== system CtrPlatform/Signal Re-group/Re-group_R5 ==
  In_R5 : Inport
  Demux2 : Demux
  Mux : Mux  Inputs=3
  JntVelAcc_R5 : Outport
  Torque_R5 : Outport  Port=2
  wires:
  In_R5/1 -> Demux2/1
  Demux2/1 -> Mux/1
  Demux2/2 -> Mux/2
  Demux2/3 -> Mux/3
  Demux2/4 -> Torque_R5/1
  Mux/1 -> JntVelAcc_R5/1

== system CtrPlatform/Signal Re-group/Re-group_R6 ==
  In_R6 : Inport
  Demux2 : Demux
  Mux : Mux  Inputs=3
  JntVelAcc_R6 : Outport
  Torque_R6 : Outport  Port=2
  wires:
  Mux/1 -> JntVelAcc_R6/1
  Demux2/4 -> Torque_R6/1
  Demux2/3 -> Mux/3
  Demux2/2 -> Mux/2
  Demux2/1 -> Mux/1
  In_R6/1 -> Demux2/1
